simulink model "controle"  (R2018b)
settings: Solver=FixedStepAuto  StartTime=0.0  StopTime=2000  FixedStep=0.01  RelTol=1e-3
libraries: neural x107, simulink x6
(part 3 of 3)

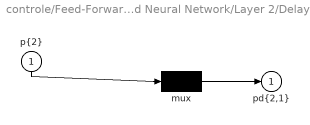
== system controle/Feed-Forward Neural Network/Layer 2/Delays 1 ==
  "p{2}" : Inport  PortDimensions=100
      mask Display: e = 0.06;c1 = [120 230 180]/255;c2 = ([120 230 180]+0)/(256+128);c3 = ([120 230 180]+128)/(256+128);patch([0 1 1 0],[0 0 1 1],c1);patch([0 1 1 1-e 1-e 0+e],[0 0 1 1-e 0+e 0+e],c2);patch([0 0 1 1-e 0+e 0+e],[0 1 1 1-e 1-e 0+e],c3);plot([0 1 1 0 0],[0 0 1 1 0]);
  mux : Mux  Inputs=1
      mask Display: e = 0.06;c1 = [120 150 230]/255;c2 = ([120 150 230]+0)/383;c3 = ([120 150 230]+128)/383;patch([0 1 1 0],[0 0 1 1],c1);patch([0 1 1 1-e 1-e 0+e],[0 0 1 1-e 0+e 0+e],c2);patch([0 0 1 1-e 0+e 0+e],[0 1 1 1-e 1-e 0+e],c3);plot([0 1 1 0 0],[0 0 1 1 0]);disp('Mux')
  "pd{2,1}" : Outport
      mask Display: e = 0.06;c1 = [120 230 180]/255;c2 = ([120 230 180]+0)/(256+128);c3 = ([120 230 180]+128)/(256+128);patch([0 1 1 0],[0 0 1 1],c1);patch([0 1 1 1-e 1-e 0+e],[0 0 1 1-e 0+e 0+e],c2);patch([0 0 1 1-e 0+e 0+e],[0 1 1 1-e 1-e 0+e],c3);plot([0 1 1 0 0],[0 0 1 1 0]);
  wires:
  mux/1 -> "pd{2,1}"/1
  "p{2}"/1 -> mux/1

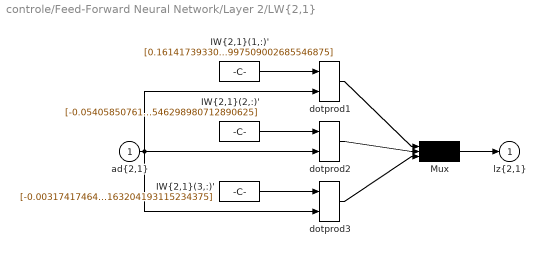
== system controle/Feed-Forward Neural Network/Layer 2/LW{2,1} ==
  "ad{2,1}" : Inport  PortDimensions=100
      mask Display: e = 0.06;c1 = [120 230 180]/255;c2 = ([120 230 180]+0)/(256+128);c3 = ([120 230 180]+128)/(256+128);patch([0 1 1 0],[0 0 1 1],c1);patch([0 1 1 1-e 1-e 0+e],[0 0 1 1-e 0+e 0+e],c2);patch([0 0 1 1-e 0+e 0+e],[0 1 1 1-e 1-e 0+e],c3);plot([0 1 1 0 0],[0 0 1 1 0]);
  "IW{2,1}(1,:)'" : Constant  Value=[0.1614173933052516496378103738607023842632770538330078125;0.391686413749836537245840872856206260621547698974609375;-0.01536981768681838951551288374730575014837086200714111328125;0.008140070097598921250448000819233129732310771942138671875;-0.045034890304621440215715466592882876284420490264892578125;-0.0162193774226591265474883840624897857196629047393798828125;-0.0967741990651240502341323690416174940764904022216796875;0.1823605603769521132928588258437230251729488372802734375;-0.062817582074687461357598294853232800960540771484375;0.013379690027190478673890794425460626371204853057861328125;-0.126159713768725867399922435652115382254123687744140625;0.12363073013000593081134326212122687138617038726806640625;0.0160505365768892176159265972046341630630195140838623046875;0.4324374285925689509468838878092356026172637939453125;0.022029375864191520772994437038505566306412220001220703125;0.0015420000649642891243917830479404074139893054962158203125;0.0281087690402712919723882123435032553970813751220703125;-0.042482325403330134516721727777621708810329437255859375;0.45546583141217666934608132578432559967041015625;0.049113755051425921072105751363778836093842983245849609375;-0.0050633144094610893493069170290254987776279449462890625;-0.02459589621085390975796514112516888417303562164306640625;-0.01017291248708471727846269772044252022169530391693115234375;0.02388641108845461491494432948456960730254650115966796875;-0.06152679525950251193666673543702927418053150177001953125;-0.0236091470629717255225177297006666776724159717559814453125;0.07502709079916396184284366199790383689105510711669921875;-0.04137093688499964005966802460534381680190563201904296875;-0.04203226536200065088788591083357459865510463714599609375;0.0344928905339884350755852437941939570009708404541015625;-0.02258934060030663715235021982152829878032207489013671875;-0.0992470166931706809787527845401200465857982635498046875;-0.05797893712215122785647025693833711557090282440185546875;-0.03657698337090810325467060692972154356539249420166015625;-0.033022133771878271757405087782899499870836734771728515625;-0.0746549503524712998459023083341890014708042144775390625;-0.052071131012503886481557202614567358978092670440673828125;-0.26418775001655159240243619933607988059520721435546875;-0.261430603585112830700154518126510083675384521484375;0.0032028353503865173400322330365952439024113118648529052734375;-0.03378473152017770486654768546941340900957584381103515625;-0.03735498722261111625986274020760902203619480133056640625;0.01555075768509141774520454504227018333040177822113037109375;0.042165773470489185947851495939175947569310665130615234375;-0.01213471847319964012912318906955988495610654354095458984375;0.04963758259371701953011069008425693027675151824951171875;0.1109251195215507912461561090822215192019939422607421875;-0.02251733480405891663078676856457605026662349700927734375;-0.1441625637462733144911197769033606164157390594482421875;-0.0188289285991417067178677058336688787676393985748291015625;-0.071689969391736274584303600931889377534389495849609375;-0.0451766764691614586268997300066985189914703369140625;-0.0838385542512379011714784837749903090298175811767578125;-0.0262939378156766927208121131798179703764617443084716796875;-0.0260367572781814889115725719648253289051353931427001953125;0.00928993622120710509093566287219800869934260845184326171875;0.1712010318900571148592604231453151442110538482666015625;0.021318812381570566294453072941905702464282512664794921875;-0.0273554434490133370483366803682656609453260898590087890625;-0.0225375143614320351537205766589977429248392581939697265625;0.057471026941569081092353599160560406744480133056640625;0.0130537233157040875874965735192745341919362545013427734375;0.0913668819460472236837489390381961129605770111083984375;-0.83337272509881776816342835445539094507694244384765625;-0.4490835964222938958556596844573505222797393798828125;-0.391091301389933698740009049288346432149410247802734375;-0.0800137515324721160236975947555038146674633026123046875 ...(+1957 chars)]
      mask Display: e = 0.06;c1 = [120 150 230]/255;c2 = ([120 150 230]+0)/383;c3 = ([120 150 230]+128)/383;patch([0 1 1 0],[0 0 1 1],c1);patch([0 1 1 1-e 1-e 0+e],[0 0 1 1-e 0+e 0+e],c2);patch([0 0 1 1-e 0+e 0+e],[0 1 1 1-e 1-e 0+e],c3);plot([0 1 1 0 0],[0 0 1 1 0]);disp('weights');
  "IW{2,1}(2,:)'" : Constant  Value=[-0.05405850761062981624238688027617172338068485260009765625;-0.469351410280861414126007957747788168489933013916015625;-0.0425055806612881503792067405811394564807415008544921875;0.011816792574272171056914970677098608575761318206787109375;0.0480134335688146840492862565952236764132976531982421875;-0.174808899339953971452388259422150440514087677001953125;-0.036921321129043775666200843943443032912909984588623046875;0.0816839138442352064028995073385885916650295257568359375;-0.090574650712231308258282069800770841538906097412109375;0.025757960762517344288635712246104958467185497283935546875;-0.0152982756645585228627570728576756664551794528961181640625;0.16985075323036868955028921845951117575168609619140625;0.0957315338681934135944828767605940811336040496826171875;-0.85744820692617695900850094403722323477268218994140625;0.050199360726880082328449361739330925047397613525390625;0.00470650745252161779863531165801759925670921802520751953125;0.0839427725116109468839198370915255509316921234130859375;-0.0257292686197341281817418945365716353990137577056884765625;-1.04109457088596446538986128871329128742218017578125;0.041315142439042086552891674955390044488012790679931640625;0.004804121978888226292270235973091985215432941913604736328125;0.09502575938584641168649369546983507461845874786376953125;0.0440776819669836950055241686641238629817962646484375;0.0305928594933899712648983637564015225507318973541259765625;0.0383528989505472761578630525036714971065521240234375;-0.01326819911336427244841207340186883811838924884796142578125;0.053534721573237076253093391642323695123195648193359375;-0.05740842896692292807170332480382057838141918182373046875;-0.004300761694933511077032495251160071347840130329132080078125;0.034396371412033492631632469738178770057857036590576171875;0.0471309965984743062250572620541788637638092041015625;-0.11517475115568269472543505571593414060771465301513671875;0.0567398127430037979568311357070342637598514556884765625;-0.03398175139662577837196266727914917282760143280029296875;-0.0282190826489212183425525637403552536852657794952392578125;-0.002265774557502951702669946598689421080052852630615234375;0.057641093702152250421999468699141289107501506805419921875;0.2482445412412614960118162343860603868961334228515625;-0.0236912479636568196195156588146346621215343475341796875;0.005926939265777308139815371390568543574772775173187255859375;0.04086176077190471767064394725821330212056636810302734375;-0.0116238296875765499682753301158300018869340419769287109375;0.001815021553354689322345993929275209666229784488677978515625;-0.00489846727936237014144893464617780409753322601318359375;2.1243397978745769995312375755247558117844164371490478515625e-05;-0.014859372636858693417227783584166900254786014556884765625;0.05529698545619075866763836302197887562215328216552734375;-0.029851991184863722883502390459398156963288784027099609375;-0.291792580014098190677174216034472920000553131103515625;-0.004710881974836530171335535754906231886707246303558349609375;0.01921561198962389027666830543239484541118144989013671875;-0.0130767677890184265410145059149726876057684421539306640625;0.032881775464514852169717329388731741346418857574462890625;-0.001312553997202886395256893337091241846792399883270263671875;-0.03336813159221778402052649425968411378562450408935546875;0.016264769672934865918367819404011243022978305816650390625;0.1480243676719637802019491346072754822671413421630859375;0.0433295268982549497405187821641447953879833221435546875;-0.0294628865527019334624725388493970967829227447509765625;-0.0186617494646469823937895426979594049043953418731689453125;0.01099464865899938727233919877335210912860929965972900390625;-0.000488348464793256394067544334802732919342815876007080078125;0.0945185519186334255348214128389372490346431732177734375;-0.66899000945319697652990953429252840578556060791015625;-0.39922848817334044557725292179384268820285797119140625;-0.270744978340045017173309815916582010686397552490234375;-0.1225091917072283764778006798223941586911678314208984375 ...(+1952 chars)]
      mask Display: e = 0.06;c1 = [120 150 230]/255;c2 = ([120 150 230]+0)/383;c3 = ([120 150 230]+128)/383;patch([0 1 1 0],[0 0 1 1],c1);patch([0 1 1 1-e 1-e 0+e],[0 0 1 1-e 0+e 0+e],c2);patch([0 0 1 1-e 0+e 0+e],[0 1 1 1-e 1-e 0+e],c3);plot([0 1 1 0 0],[0 0 1 1 0]);disp('weights');
  "IW{2,1}(3,:)'" : Constant  Value=[-0.00317417464995305674546610674724433920346200466156005859375;-0.594203557022984885094274432049132883548736572265625;0.058272002295495506363209869959973730146884918212890625;0.074518725659414031259331068213214166462421417236328125;0.008806279539039167658653894932285766117274761199951171875;0.343101495826379443432330162977450527250766754150390625;0.1278414660550616643863719446017057634890079498291015625;0.0948018636307593476342248095534159801900386810302734375;0.0807954637592410429558498208280070684850215911865234375;-0.0174811255558408283616866896181818447075784206390380859375;0.24840070796241142669913415375049225986003875732421875;0.120873531840177517171497356684994883835315704345703125;-0.101730934343692236421219377007219009101390838623046875;-0.259593837570720353813413794341613538563251495361328125;-0.0212159030958661565247069802353507839143276214599609375;0.000973402192628970881760341882227294263429939746856689453125;-0.127778720464549966351341936388052999973297119140625;-0.00198974462648156789901232599504510289989411830902099609375;-0.1730847456537477346838471703449613414704799652099609375;-0.05862490777655425533421151840229867957532405853271484375;0.04755172495406057020517209821264259517192840576171875;0.004907777624886235090517772050588973797857761383056640625;-0.0036145468115950478427134129333353484980762004852294921875;0.024933808922340705560571905152755789458751678466796875;-0.1485041357202992184927126118054729886353015899658203125;0.0142497215682911397560683752772092702798545360565185546875;-0.10984019245161015521095038138810195960104465484619140625;0.0638320394321995332465036199209862388670444488525390625;0.06545579480268938488141117204577312804758548736572265625;-0.08841537606391376702408280152667430229485034942626953125;-0.1018615323221314372670320835823076777160167694091796875;0.022860474967382297950546643505731481127440929412841796875;-0.0673044986677250045570275460704579018056392669677734375;0.001997409198017600917562930362691986374557018280029296875;0.0158975254934923260208279316429980099201202392578125;0.1451095585843932556091573360390611924231052398681640625;-0.0288567253180988352034841426529965247027575969696044921875;-0.225638754629068516432965907370089553296566009521484375;0.392835211086278224268397707419353537261486053466796875;0.002362439937312554860682212165556848049163818359375;-0.0215714241196658662591545407849480397999286651611328125;0.05028617083451179803343933372161700390279293060302734375;-0.0245076269527397909431254419132528710179030895233154296875;-0.07140809875189442490484026393460226245224475860595703125;-0.000403236063546780101711497490413194100256077945232391357421875;-0.00449186663935896048072127229033867479301989078521728515625;0.058164240929808819213775450407410971820354461669921875;0.0159647293734709073975697180003407993353903293609619140625;-0.259777856072183954694310159538872539997100830078125;0.0644775867171562822033337170068989507853984832763671875;-0.0457515508198112763604825659058406017720699310302734375;0.07315612881064714745349419899866916239261627197265625;0.1240466498040135590041899149582604877650737762451171875;0.003190087716531113393170215886129881255328655242919921875;0.00523446147176048932891934128974753548391163349151611328125;0.08540155710166140445860349927897914312779903411865234375;-0.25170504407930971435547462533577345311641693115234375;-0.04873136884470087581977537638522335328161716461181640625;0.037862724190693648751437905275452067144215106964111328125;0.0247022563484389952315201099963815067894756793975830078125;-0.001908500382908043420393529032708102022297680377960205078125;0.0200219284216452790559070962217447231523692607879638671875;-0.18889184311003781591153938279603607952594757080078125;-0.8122464864022942432342233587405644357204437255859375;-0.395645659022789752956583697596215642988681793212890625;-0.373588419561301510185558072407729923725128173828125;0.1391875506580743937501409845935995690524578094482421875 ...(+1940 chars)]
      mask Display: e = 0.06;c1 = [120 150 230]/255;c2 = ([120 150 230]+0)/383;c3 = ([120 150 230]+128)/383;patch([0 1 1 0],[0 0 1 1],c1);patch([0 1 1 1-e 1-e 0+e],[0 0 1 1-e 0+e 0+e],c2);patch([0 0 1 1-e 0+e 0+e],[0 1 1 1-e 1-e 0+e],c3);plot([0 1 1 0 0],[0 0 1 1 0]);disp('weights');
  Mux : Mux  Inputs=3
      mask Display: e = 0.06;c1 = [120 150 230]/255;c2 = ([120 150 230]+0)/383;c3 = ([120 150 230]+128)/383;patch([0 1 1 0],[0 0 1 1],c1);patch([0 1 1 1-e 1-e 0+e],[0 0 1 1-e 0+e 0+e],c2);patch([0 0 1 1-e 0+e 0+e],[0 1 1 1-e 1-e 0+e],c3);plot([0 1 1 0 0],[0 0 1 1 0]);disp('Mux');
  dotprod1 : neural/Weight Functions/dotprod
  dotprod2 : neural/Weight Functions/dotprod
  dotprod3 : neural/Weight Functions/dotprod
  "lz{2,1}" : Outport
      mask Display: e = 0.06;c1 = [120 230 180]/255;c2 = ([120 230 180]+0)/(256+128);c3 = ([120 230 180]+128)/(256+128);patch([0 1 1 0],[0 0 1 1],c1);patch([0 1 1 1-e 1-e 0+e],[0 0 1 1-e 0+e 0+e],c2);patch([0 0 1 1-e 0+e 0+e],[0 1 1 1-e 1-e 0+e],c3);plot([0 1 1 0 0],[0 0 1 1 0]);
  wires:
  Mux/1 -> "lz{2,1}"/1
  dotprod3/1 -> Mux/3
  "IW{2,1}(3,:)'"/1 -> dotprod3/1
  dotprod2/1 -> Mux/2
  "IW{2,1}(2,:)'"/1 -> dotprod2/1
  dotprod1/1 -> Mux/1
  "ad{2,1}"/1 -> dotprod3/2, dotprod2/2, dotprod1/2
  "IW{2,1}(1,:)'"/1 -> dotprod1/1

== matlab function controle/camera ==
  data: input input; x output; output input; y output; z output
function [x,y,z] = camera(input, output)
x = input(1) - output(1);
y = input(2) - output(2);
z = input(3) - output(3);
end
